simulink model "sl_pigle_Population2020"  (R2020a)
settings: Solver=FixedStepAuto  StartTime=0.0  StopTime=params.stop_time  FixedStep=params.sample_time  RelTol=1e-3  EnableMultiTasking=on
PreLoadFcn:
  | load pigle_data.mat
InitFcn:
  | load pigle_data.mat
undefined symbols (not defined in the file or in its folder): DiscIntNeverNeededParam, params
libraries: simulink x7, dspmtrx3 x2
(part 2 of 2)

== system sl_pigle_Population2020/Population/Population 0/Delta R/dtheta/Subsystem1/For Each Subsystem1/Subsystem1 ==
  theta : Inport
  Constant : Constant  Value=0
  Constant1 : Constant
  If : If  IfExpression=u1==0
  If Action Subsystem : Subsystem  TreatAsAtomicUnit=on
  If Action Subsystem1 : Subsystem  TreatAsAtomicUnit=on
  Merge : Merge
  Out1 : Outport
  wires:
  If/1 -> If Action Subsystem/Action
  If Action Subsystem/1(Out1) -> Merge/1
  Merge/1 -> Out1/1
  If Action Subsystem1/1(Out1) -> Merge/2
  Constant/1 -> If Action Subsystem/1(In1)
  If/2 -> If Action Subsystem1/Action
  theta/1 -> If/1
  Constant1/1 -> If Action Subsystem1/1(In1)

== system sl_pigle_Population2020/Population/Population 0/Delta R/dtheta/Subsystem1/Subsystem1/For Iterator Subsystem ==
  sintilt : Inport
  Natoms : Inport  Port=2
  For Iterator : ForIterator  IterationSource=external
  Selector1 : Selector  NumberOfDimensions=2  InputPortWidth=2  IndexOptions=Select all,Index vector (port)  Indices=1:params.prtcl(1).momenta_dimension_theta,1:params.prtcl(1).Nprtcl  OutputSizes=1,1
  Subsystem1 : Subsystem
  Out1 : Outport
  wires:
  Natoms/1 -> For Iterator/1
  Subsystem1/1(Out1) -> Out1/1
  sintilt/1 -> Selector1/1
  Selector1/1 -> Subsystem1/2(sintilt), Subsystem1/1(sin2)
  For Iterator/1 -> Selector1/2

== system sl_pigle_Population2020/Population/Population 0/Delta R/dtheta/Subsystem1/Subsystem1/If Action Subsystem ==
  In1 : Inport
  Action Port : ActionPort
  Out1 : Outport
  wires:
  In1/1 -> Out1/1

== system sl_pigle_Population2020/Population/Population 0/Delta R/dtheta/Subsystem1/Subsystem1/If Action Subsystem1 ==
  In1 : Inport
  Action Port : ActionPort
  Out1 : Outport
  wires:
  In1/1 -> Out1/1

== system sl_pigle_Population2020/Population/Population 0/Delta R/dtheta/Subsystem1/Subsystem1/If Action Subsystem2 ==
  In1 : Inport
  Action Port : ActionPort
  Out1 : Outport
  wires:
  In1/1 -> Out1/1

== system sl_pigle_Population2020/Population/Population 0/Delta R/dtheta/Subsystem1/Subsystem1/If Action Subsystem3 ==
  In1 : Inport
  Action Port : ActionPort
  For Each Subsystem : Subsystem  TreatAsAtomicUnit=on
  Out1 : Outport
  wires:
  In1/1 -> For Each Subsystem/1(sin2)
  For Each Subsystem/1(Out1) -> Out1/1

== system sl_pigle_Population2020/Population/Population 0/Delta R/dtheta/Subsystem1/Subsystem2/For Iterator Subsystem ==
  sintilt : Inport
  Natoms : Inport  Port=2
  For Iterator : ForIterator  IterationSource=external
  Selector1 : Selector  NumberOfDimensions=2  InputPortWidth=2  IndexOptions=Select all,Index vector (port)  Indices=1:params.prtcl(1).momenta_dimension_theta,1:params.prtcl(1).Nprtcl  OutputSizes=1,1
  Subsystem1 : Subsystem
  Out1 : Outport
  wires:
  Natoms/1 -> For Iterator/1
  Subsystem1/1(Out1) -> Out1/1
  sintilt/1 -> Selector1/1
  Selector1/1 -> Subsystem1/2(sintilt), Subsystem1/1(sin2)
  For Iterator/1 -> Selector1/2

== system sl_pigle_Population2020/Population/Population 0/Delta R/dtheta/Subsystem1/Subsystem2/If Action Subsystem ==
  In1 : Inport
  Action Port : ActionPort
  Out1 : Outport
  wires:
  In1/1 -> Out1/1

== system sl_pigle_Population2020/Population/Population 0/Delta R/dtheta/Subsystem1/Subsystem2/If Action Subsystem1 ==
  In1 : Inport
  Action Port : ActionPort
  Out1 : Outport
  wires:
  In1/1 -> Out1/1

== system sl_pigle_Population2020/Population/Population 0/Delta R/dtheta/Subsystem1/Subsystem2/If Action Subsystem2 ==
  In1 : Inport
  Action Port : ActionPort
  Out1 : Outport
  wires:
  In1/1 -> Out1/1

== system sl_pigle_Population2020/Population/Population 0/Delta R/dtheta/Subsystem1/Subsystem2/If Action Subsystem3 ==
  In1 : Inport
  Action Port : ActionPort
  For Each Subsystem : Subsystem  TreatAsAtomicUnit=on
  Out1 : Outport
  wires:
  In1/1 -> For Each Subsystem/1(sin2)
  For Each Subsystem/1(Out1) -> Out1/1

== system sl_pigle_Population2020/Population/Population 0/Delta R/dtilt/Subsystem/For Iterator Subsystem/Subsystem1 ==
  sin2 : Inport
  sintilt : Inport  Port=2
  Constant : Constant
  If : If  NumInputs=2  IfExpression=u1==0
  If Action Subsystem : Subsystem  TreatAsAtomicUnit=on
  If Action Subsystem1 : Subsystem  TreatAsAtomicUnit=on
  Merge : Merge
  Out1 : Outport
  wires:
  If/1 -> If Action Subsystem/Action
  If Action Subsystem/1(Out1) -> Merge/1
  Merge/1 -> Out1/1
  If Action Subsystem1/1(Out1) -> Merge/2
  Constant/1 -> If Action Subsystem/1(In1)
  If/2 -> If Action Subsystem1/Action
  sin2/1 -> If/1
  sintilt/1 -> If Action Subsystem1/1(In1)

== system sl_pigle_Population2020/Population/Population 0/Delta R/dtilt/Subsystem/If Action Subsystem3/For Each Subsystem ==
  sin2 : Inport  Partition=on  PartitionDimension=2  PartitionWidth=1  PartitionOffset=0
  For Each : ForEach  DisableCoverage=on
  Subsystem1 : Subsystem
  Out1 : Outport  ConcatenationDimension=1
  wires:
  sin2/1 -> Subsystem1/1(sin2), Subsystem1/2(sintilt)
  Subsystem1/1(Out1) -> Out1/1

== system sl_pigle_Population2020/Population/Population 0/Delta R/dtheta/Subsystem1/For Each Subsystem/Subsystem1/If Action Subsystem ==
  In1 : Inport
  Action Port : ActionPort
  Out1 : Outport
  wires:
  In1/1 -> Out1/1

== system sl_pigle_Population2020/Population/Population 0/Delta R/dtheta/Subsystem1/For Each Subsystem/Subsystem1/If Action Subsystem1 ==
  In1 : Inport
  Action Port : ActionPort
  Out1 : Outport
  wires:
  In1/1 -> Out1/1

== system sl_pigle_Population2020/Population/Population 0/Delta R/dtheta/Subsystem1/For Each Subsystem1/Subsystem1/If Action Subsystem ==
  In1 : Inport
  Action Port : ActionPort
  Out1 : Outport
  wires:
  In1/1 -> Out1/1

== system sl_pigle_Population2020/Population/Population 0/Delta R/dtheta/Subsystem1/For Each Subsystem1/Subsystem1/If Action Subsystem1 ==
  In1 : Inport
  Action Port : ActionPort
  Out1 : Outport
  wires:
  In1/1 -> Out1/1

== system sl_pigle_Population2020/Population/Population 0/Delta R/dtheta/Subsystem1/Subsystem1/For Iterator Subsystem/Subsystem1 ==
  sin2 : Inport
  sintilt : Inport  Port=2
  Constant : Constant
  If : If  NumInputs=2  IfExpression=u1==0
  If Action Subsystem : Subsystem  TreatAsAtomicUnit=on
  If Action Subsystem1 : Subsystem  TreatAsAtomicUnit=on
  Merge : Merge
  Out1 : Outport
  wires:
  If/1 -> If Action Subsystem/Action
  If Action Subsystem/1(Out1) -> Merge/1
  Merge/1 -> Out1/1
  If Action Subsystem1/1(Out1) -> Merge/2
  Constant/1 -> If Action Subsystem/1(In1)
  If/2 -> If Action Subsystem1/Action
  sin2/1 -> If/1
  sintilt/1 -> If Action Subsystem1/1(In1)

== system sl_pigle_Population2020/Population/Population 0/Delta R/dtheta/Subsystem1/Subsystem1/If Action Subsystem3/For Each Subsystem ==
  sin2 : Inport  Partition=on  PartitionDimension=2  PartitionWidth=1  PartitionOffset=0
  For Each : ForEach  DisableCoverage=on
  Subsystem1 : Subsystem
  Out1 : Outport  ConcatenationDimension=1
  wires:
  sin2/1 -> Subsystem1/1(sin2), Subsystem1/2(sintilt)
  Subsystem1/1(Out1) -> Out1/1

== system sl_pigle_Population2020/Population/Population 0/Delta R/dtheta/Subsystem1/Subsystem2/For Iterator Subsystem/Subsystem1 ==
  sin2 : Inport
  sintilt : Inport  Port=2
  Constant : Constant
  If : If  NumInputs=2  IfExpression=u1==0
  If Action Subsystem : Subsystem  TreatAsAtomicUnit=on
  If Action Subsystem1 : Subsystem  TreatAsAtomicUnit=on
  Merge : Merge
  Out1 : Outport
  wires:
  If/1 -> If Action Subsystem/Action
  If Action Subsystem/1(Out1) -> Merge/1
  Merge/1 -> Out1/1
  If Action Subsystem1/1(Out1) -> Merge/2
  Constant/1 -> If Action Subsystem/1(In1)
  If/2 -> If Action Subsystem1/Action
  sin2/1 -> If/1
  sintilt/1 -> If Action Subsystem1/1(In1)

== system sl_pigle_Population2020/Population/Population 0/Delta R/dtheta/Subsystem1/Subsystem2/If Action Subsystem3/For Each Subsystem ==
  sin2 : Inport  Partition=on  PartitionDimension=2  PartitionWidth=1  PartitionOffset=0
  For Each : ForEach  DisableCoverage=on
  Subsystem1 : Subsystem
  Out1 : Outport  ConcatenationDimension=1
  wires:
  sin2/1 -> Subsystem1/1(sin2), Subsystem1/2(sintilt)
  Subsystem1/1(Out1) -> Out1/1

== system sl_pigle_Population2020/Population/Population 0/Delta R/dtilt/Subsystem/For Iterator Subsystem/Subsystem1/If Action Subsystem ==
  In1 : Inport
  Action Port : ActionPort
  Out1 : Outport
  wires:
  In1/1 -> Out1/1

== system sl_pigle_Population2020/Population/Population 0/Delta R/dtilt/Subsystem/For Iterator Subsystem/Subsystem1/If Action Subsystem1 ==
  In1 : Inport
  Action Port : ActionPort
  Out1 : Outport
  wires:
  In1/1 -> Out1/1

== system sl_pigle_Population2020/Population/Population 0/Delta R/dtilt/Subsystem/If Action Subsystem3/For Each Subsystem/Subsystem1 ==
  sin2 : Inport
  sintilt : Inport  Port=2
  Constant : Constant
  If : If  IfExpression=u1==0
  If Action Subsystem : Subsystem  TreatAsAtomicUnit=on
  If Action Subsystem1 : Subsystem  TreatAsAtomicUnit=on
  Merge : Merge
  Out1 : Outport
  wires:
  If/1 -> If Action Subsystem/Action
  If Action Subsystem/1(Out1) -> Merge/1
  Merge/1 -> Out1/1
  If Action Subsystem1/1(Out1) -> Merge/2
  Constant/1 -> If Action Subsystem/1(In1)
  If/2 -> If Action Subsystem1/Action
  sin2/1 -> If/1
  sintilt/1 -> If Action Subsystem1/1(In1)

== system sl_pigle_Population2020/Population/Population 0/Delta R/dtheta/Subsystem1/Subsystem1/For Iterator Subsystem/Subsystem1/If Action Subsystem ==
  In1 : Inport
  Action Port : ActionPort
  Out1 : Outport
  wires:
  In1/1 -> Out1/1

== system sl_pigle_Population2020/Population/Population 0/Delta R/dtheta/Subsystem1/Subsystem1/For Iterator Subsystem/Subsystem1/If Action Subsystem1 ==
  In1 : Inport
  Action Port : ActionPort
  Out1 : Outport
  wires:
  In1/1 -> Out1/1

== system sl_pigle_Population2020/Population/Population 0/Delta R/dtheta/Subsystem1/Subsystem1/If Action Subsystem3/For Each Subsystem/Subsystem1 ==
  sin2 : Inport
  sintilt : Inport  Port=2
  Constant : Constant
  If : If  IfExpression=u1==0
  If Action Subsystem : Subsystem  TreatAsAtomicUnit=on
  If Action Subsystem1 : Subsystem  TreatAsAtomicUnit=on
  Merge : Merge
  Out1 : Outport
  wires:
  If/1 -> If Action Subsystem/Action
  If Action Subsystem/1(Out1) -> Merge/1
  Merge/1 -> Out1/1
  If Action Subsystem1/1(Out1) -> Merge/2
  Constant/1 -> If Action Subsystem/1(In1)
  If/2 -> If Action Subsystem1/Action
  sin2/1 -> If/1
  sintilt/1 -> If Action Subsystem1/1(In1)

== system sl_pigle_Population2020/Population/Population 0/Delta R/dtheta/Subsystem1/Subsystem2/For Iterator Subsystem/Subsystem1/If Action Subsystem ==
  In1 : Inport
  Action Port : ActionPort
  Out1 : Outport
  wires:
  In1/1 -> Out1/1

== system sl_pigle_Population2020/Population/Population 0/Delta R/dtheta/Subsystem1/Subsystem2/For Iterator Subsystem/Subsystem1/If Action Subsystem1 ==
  In1 : Inport
  Action Port : ActionPort
  Out1 : Outport
  wires:
  In1/1 -> Out1/1

== system sl_pigle_Population2020/Population/Population 0/Delta R/dtheta/Subsystem1/Subsystem2/If Action Subsystem3/For Each Subsystem/Subsystem1 ==
  sin2 : Inport
  sintilt : Inport  Port=2
  Constant : Constant
  If : If  IfExpression=u1==0
  If Action Subsystem : Subsystem  TreatAsAtomicUnit=on
  If Action Subsystem1 : Subsystem  TreatAsAtomicUnit=on
  Merge : Merge
  Out1 : Outport
  wires:
  If/1 -> If Action Subsystem/Action
  If Action Subsystem/1(Out1) -> Merge/1
  Merge/1 -> Out1/1
  If Action Subsystem1/1(Out1) -> Merge/2
  Constant/1 -> If Action Subsystem/1(In1)
  If/2 -> If Action Subsystem1/Action
  sin2/1 -> If/1
  sintilt/1 -> If Action Subsystem1/1(In1)

== system sl_pigle_Population2020/Population/Population 0/Delta R/dtilt/Subsystem/If Action Subsystem3/For Each Subsystem/Subsystem1/If Action Subsystem ==
  In1 : Inport
  Action Port : ActionPort
  Out1 : Outport
  wires:
  In1/1 -> Out1/1

== system sl_pigle_Population2020/Population/Population 0/Delta R/dtilt/Subsystem/If Action Subsystem3/For Each Subsystem/Subsystem1/If Action Subsystem1 ==
  In1 : Inport
  Action Port : ActionPort
  Out1 : Outport
  wires:
  In1/1 -> Out1/1

== system sl_pigle_Population2020/Population/Population 0/Delta R/dtheta/Subsystem1/Subsystem1/If Action Subsystem3/For Each Subsystem/Subsystem1/If Action Subsystem ==
  In1 : Inport
  Action Port : ActionPort
  Out1 : Outport
  wires:
  In1/1 -> Out1/1

== system sl_pigle_Population2020/Population/Population 0/Delta R/dtheta/Subsystem1/Subsystem1/If Action Subsystem3/For Each Subsystem/Subsystem1/If Action Subsystem1 ==
  In1 : Inport
  Action Port : ActionPort
  Out1 : Outport
  wires:
  In1/1 -> Out1/1

== system sl_pigle_Population2020/Population/Population 0/Delta R/dtheta/Subsystem1/Subsystem2/If Action Subsystem3/For Each Subsystem/Subsystem1/If Action Subsystem ==
  In1 : Inport
  Action Port : ActionPort
  Out1 : Outport
  wires:
  In1/1 -> Out1/1

== system sl_pigle_Population2020/Population/Population 0/Delta R/dtheta/Subsystem1/Subsystem2/If Action Subsystem3/For Each Subsystem/Subsystem1/If Action Subsystem1 ==
  In1 : Inport
  Action Port : ActionPort
  Out1 : Outport
  wires:
  In1/1 -> Out1/1
